simulink model "robot_leg_opt"  (R2015b)
settings: Solver=ode23t  StartTime=0.0  StopTime=2  MaxStep=0.05  RelTol=1e-3
values from neighbouring files (symbols this model uses):
  B0 = q(3)    [costFunc.m]    (also in leg_mechanical_params.m = 3266.28463902)
  DamperStrokeMax = 0.1    [leg_mechanical_params.m]
  dthetaHd = 0    [leg_mechanical_params.m]
  dthetaKd = 0    [leg_mechanical_params.m]
  Hd_knee = 5*0    (= 0)    [leg_mechanical_params.m]
  Hp_knee = 50*0    (= 0)    [leg_mechanical_params.m]
  k_gx = (2*(m_F+m_S+m_T)+m_HAT)*g/0.1    (= 7848)    [leg_mechanical_params.m]
  k_gy = (2*(m_F+m_S+m_T)+m_HAT)*g/0.01    (= 78480)    [leg_mechanical_params.m]
  kap0 = 0    [leg_mechanical_params.m]
  Kd_knee = q(2)    [costFunc.m]    (also in leg_mechanical_params.m = 7.0905816766)
  Kp_knee = q(1)    [costFunc.m]    (also in leg_mechanical_params.m = 4034.50740334)
  LBtnShin = 0    [leg_mechanical_params.m]
  LMidShin = 0    [leg_mechanical_params.m]
  lspring0 = 0.5582    [leg_mechanical_params.m]
  mu_slide = 0.8    [leg_mechanical_params.m]
  mu_stick = 0.9    [leg_mechanical_params.m]
  thetaHd = thetaH0    (= 0.785398163397)    [leg_mechanical_params.m]
  thetaKd = thetaK0    (= -1.0471975512)    [leg_mechanical_params.m]
  v_gx_max = 0.03    [leg_mechanical_params.m]
  v_gy_max = 0.03    [leg_mechanical_params.m]
  vLimit = 0.01    [leg_mechanical_params.m]
  Y0 = 3    [initLegModel.m]
undefined symbols (not defined in the file or in its folder): sgn, t_friction, X, Y, Z
libraries: sm_lib x123, nesl_utility x25, fl_lib x10, simulink x8, simulink_extras x2, dspswit3 x1, HILeg_Lib x1, sm_double_wishbone_suspension_lib x1
(part 1 of 4)
settings Model: Creator=rshum  LastModifiedBy=rshum
settings DataIOCC: SaveFormat=Array
settings DebuggingCC: SolverPrmCheckMsg=warning
settings HardwareCC: ProdBitPerPointer=32  ProdLargestAtomicFloat=None  ProdIntDivRoundTo=Undefined  ProdEndianess=Unspecified  ProdWordSize=32  ProdHWDeviceType=32-bit Generic
settings GRTTargetCC: GeneratePreprocessorConditionals=Disable all
settings ConfigComp: CovModelRefEnable=Off  CovSFcnEnable=off

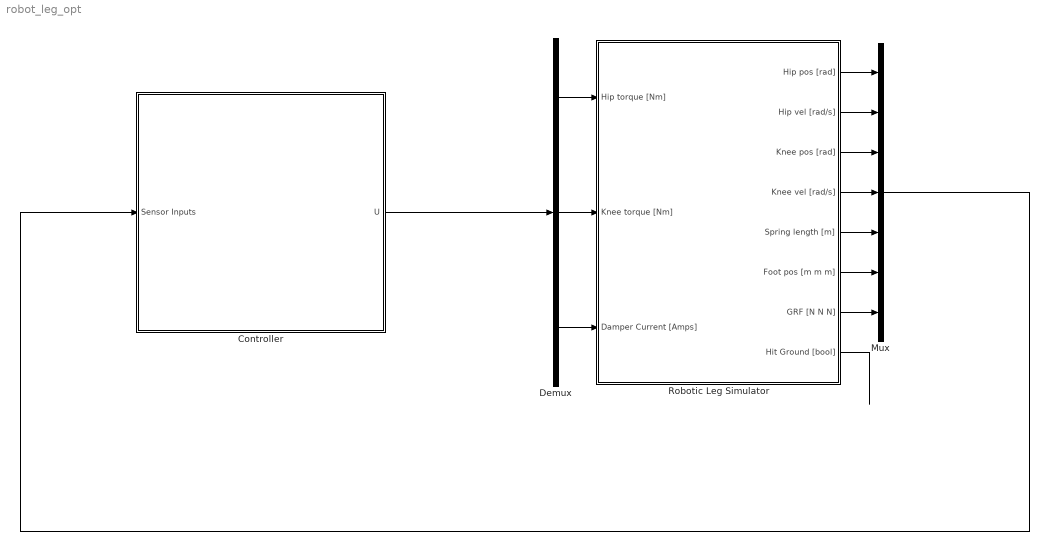
== system robot_leg_opt ==
  Controller : Subsystem
  Demux : Demux  Outputs=3
  Mux : Mux  Inputs=7
  Robotic Leg Simulator : Subsystem
  wires:
  Robotic Leg Simulator/5(Spring length [m]) -> Mux/5
  Demux/3 -> Robotic Leg Simulator/3(Damper Current [Amps])
  Robotic Leg Simulator/1(Hip pos [rad]) -> Mux/1
  Robotic Leg Simulator/2(Hip vel [rad/s]) -> Mux/2
  Robotic Leg Simulator/3(Knee pos [rad]) -> Mux/3
  Robotic Leg Simulator/4(Knee vel [rad/s]) -> Mux/4
  Mux/1 -> Controller/1(Sensor Inputs)
  Demux/1 -> Robotic Leg Simulator/1(Hip torque [Nm])
  Demux/2 -> Robotic Leg Simulator/2(Knee torque [Nm])
  Controller/1(U) -> Demux/1
  Robotic Leg Simulator/6(Foot pos [m m m]) -> Mux/6
  Robotic Leg Simulator/7(GRF [N N N]) -> Mux/7
  Robotic Leg Simulator/8(Hit Ground [bool]) -> ?

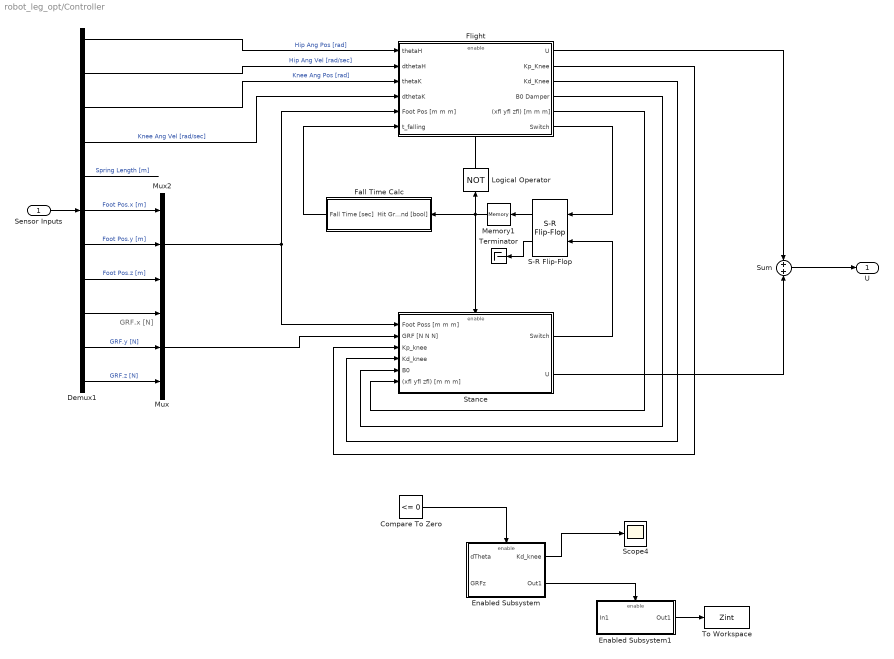
== system robot_leg_opt/Controller ==
  note: GRF.x
      | [N]
  Sensor Inputs : Inport
  Compare To Zero : simulink/Logic and Bit Operations/Compare To Zero  relop=<=  OutDataTypeStr=boolean
  Demux1 : Demux  Outputs=11
  Enabled Subsystem : Subsystem  TreatAsAtomicUnit=on
  Enabled Subsystem1 : Subsystem  TreatAsAtomicUnit=on
  Fall Time Calc : Subsystem
  Flight : Subsystem  TreatAsAtomicUnit=on
  Logical Operator : Logic  Operator=NOT  AllPortsSameDT=off  OutDataTypeStr=boolean
  Memory1 : Memory  X0=1
  Mux : Mux  Inputs=3
  Mux2 : Mux  Inputs=3
  S-R Flip-Flop : simulink_extras/Flip Flops/S-R Flip-Flop  initial_condition=1
  Scope4 : Scope
  Stance : Subsystem  TreatAsAtomicUnit=on
  Sum : Sum
  Terminator : Terminator
  To Workspace : ToWorkspace  VariableName=Zint  SampleTime=-1
      settings: MaxDataPoints=1
  U : Outport
  wires:
  Sensor Inputs/1 -> Demux1/1
  Compare To Zero/1 -> Enabled Subsystem/Enable
  Enabled Subsystem/1(Kd_knee) -> Scope4/1
  Mux/1 -> Stance/2(GRF [N N N])
  Demux1/11 -> Mux/3  "GRF.z [N]"
  Demux1/10 -> Mux/2  "GRF.y [N]"
  Demux1/9 -> Mux/1
  Enabled Subsystem/2(Out1) -> Enabled Subsystem1/Enable
  Enabled Subsystem1/1(Out1) -> To Workspace/1
  Flight/6(Switch) -> S-R Flip-Flop/1
  S-R Flip-Flop/1 -> Memory1/1
  Memory1/1 -> Stance/Enable, Fall Time Calc/1(Hit Ground [bool]), Logical Operator/1
  Stance/1(Switch) -> S-R Flip-Flop/2
  S-R Flip-Flop/2 -> Terminator/1
  Logical Operator/1 -> Flight/Enable
  Mux2/1 -> Flight/5(Foot Pos [m m m]), Stance/1(Foot Poss [m m m])
  Demux1/2 -> Flight/2(dthetaH)  "Hip Ang Vel [rad/sec]"
  Demux1/1 -> Flight/1(thetaH)  "Hip Ang Pos [rad]"
  Demux1/8 -> Mux2/3  "Foot Pos.z [m]"
  Demux1/7 -> Mux2/2  "Foot Pos.y [m]"
  Demux1/6 -> Mux2/1  "Foot Pos.x [m]"
  Demux1/5 -> ?  "Spring Length [m]"
  Demux1/4 -> Flight/4(dthetaK)  "Knee Ang Vel [rad/sec]"
  Demux1/3 -> Flight/3(thetaK)  "Knee Ang Pos [rad]"
  Fall Time Calc/1(Fall Time [sec]) -> Flight/6(t_falling)
  Flight/5((xfl yfl zfl) [m m m]) -> Stance/6((xfl yfl zfl) [m m m])
  Flight/4(B0 Damper) -> Stance/5(B0)
  Flight/3(Kd_Knee) -> Stance/4(Kd_knee)
  Flight/2(Kp_Knee) -> Stance/3(Kp_knee)
  Sum/1 -> U/1
  Flight/1(U) -> Sum/1
  Stance/2(U) -> Sum/2

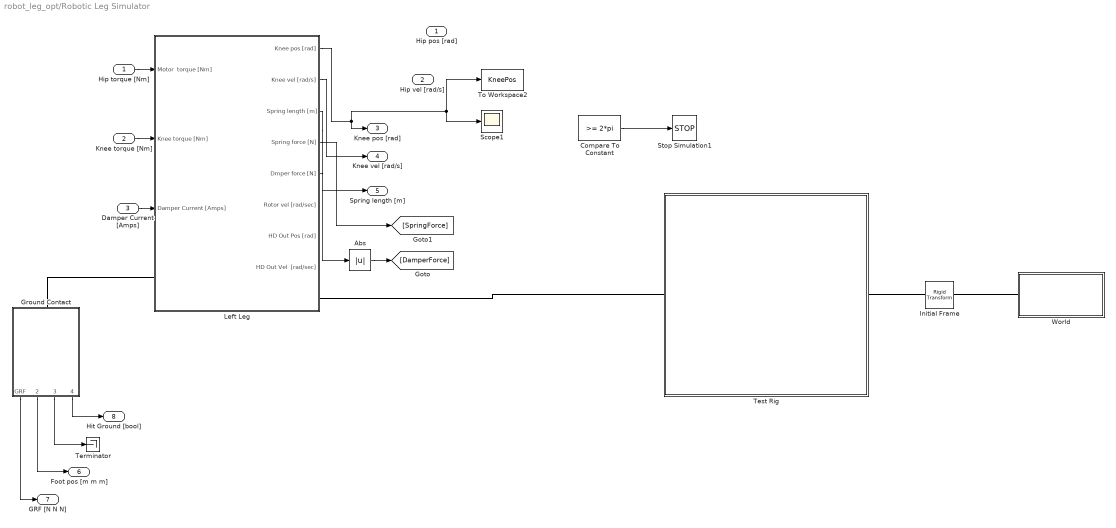
== system robot_leg_opt/Robotic Leg Simulator ==
  Hip torque [Nm] : Inport
  Knee torque [Nm] : Inport  Port=2
  Damper Current [Amps] : Inport  Port=3
  Abs : Abs
  Compare To Constant : simulink/Logic and Bit Operations/Compare To Constant  relop=>=  const=2*pi  OutDataTypeStr=boolean
  Ground Contact : Subsystem  AncestorBlock=HILeg_Lib/Ground Contact  SystemSampleTime=t_friction
  Initial Frame : sm_lib/Frames and Transforms/Rigid Transform  TranslationMethod=Cartesian  TranslationLengthUnit=m  TranslationStandardAxis=+Z  TranslationStandardOffset=0  TranslationCartesianOffset=[0 0 0]  TranslationROffset=0  TranslationROffsetUnits=m  TranslationZOffset=0  TranslationZOffsetUnits=m  TranslationThetaOffset=0  TranslationThetaOffsetUnits=deg  RotationMethod=None  RotationAngleUnits=deg  RotationStandardAxis=+Z  RotationAngle=0  RotationArbitraryAxis=[0 0 1]  FollAlignAxisA=+Z  BaseAlignAxisA=+Y  FollAlignAxisB=+X  BaseAlignAxisB=+X  RotationSequenceAxes=FollowerAxes  RotationSequence=XYX  RotationSequenceAngles=[0 0 0]  RotationSequenceAnglesUnits=deg  RotationMatrix=[1 0 0; 0 1 0; 0 0 1]  BlockFunction=simmechanics.library.frames_transforms.rigid_transform
  Left Leg : Subsystem
  Scope1 : Scope
  Stop Simulation1 : Stop
  Terminator : Terminator
  Test Rig : Subsystem
      mask Display:
      | image(imread('Images/test_rig.JPG'))
      | port_label('rconn',1,'fixture')
      | port_label('lconn',1,'ground')
  To Workspace2 : ToWorkspace  VariableName=KneePos  SampleTime=-1
  World : Subsystem
  Hip pos [rad] : Outport
  Hip vel [rad/s] : Outport  Port=2
  Knee pos [rad] : Outport  Port=3
  Knee vel [rad/s] : Outport  Port=4
  Spring length [m] : Outport  Port=5
  Foot pos [m m m] : Outport  Port=6
  GRF [N N N] : Outport  Port=7
  Hit Ground [bool] : Outport  Port=8
  wires:
  Knee torque [Nm]/1 -> Left Leg/2(Knee torque [Nm])
  Left Leg/1(Knee pos [rad]) -> To Workspace2/1, Scope1/1, Knee pos [rad]/1
  Damper Current [Amps]/1 -> Left Leg/3(Damper Current [Amps])
  ? -> Hip vel [rad/s]/1
  Left Leg/3(Spring length [m]) -> Spring length [m]/1
  Hip torque [Nm]/1 -> Left Leg/1(Motor  torque [Nm])
  Left Leg/5(Dmper force [N]) -> Abs/1
  Left Leg/2(Knee vel [rad/s]) -> Knee vel [rad/s]/1
  Compare To Constant/1 -> Stop Simulation1/1
  Ground Contact/2(POS [m,m,m]) -> Foot pos [m m m]/1
  ? -> Hip pos [rad]/1
  Ground Contact/1(GRF) -> GRF [N N N]/1
  Ground Contact/4(Hit Ground [bool]) -> Hit Ground [bool]/1
  Ground Contact/3(Vel [m,m,m]) -> Terminator/1
  Abs/1 -> [DamperForce]
  Left Leg/4(Spring force [N]) -> [SpringForce]
  connections:
  Initial Frame/LConn1 -- World/LConn1
  Test Rig/LConn1 -- Initial Frame/RConn1
  Ground Contact/LConn1 -- Left Leg/LConn1
  Test Rig/RConn1 -- Left Leg/RConn1

== system robot_leg_opt/Controller/Enabled Subsystem ==
  dTheta : Inport
  GRFz : Inport  Port=2
  Enable : EnablePort
  Constant : Constant
  Gain : Gain  Gain=-1/100
  Sum : Sum  Inputs=|++
  Kd_knee : Outport  OutputWhenDisabled=reset  InitialOutput=0
  Out1 : Outport  Port=2  InitialOutput=0
  wires:
  dTheta/1 -> Sum/1
  Sum/1 -> Gain/1
  GRFz/1 -> Sum/2
  Gain/1 -> Kd_knee/1
  Constant/1 -> Out1/1

== system robot_leg_opt/Controller/Enabled Subsystem1 ==
  In1 : Inport
  Enable : EnablePort
  Abs : Abs
  Integrator : Integrator
  Out1 : Outport
  wires:
  In1/1 -> Abs/1
  Integrator/1 -> Out1/1
  Abs/1 -> Integrator/1

== system robot_leg_opt/Controller/Fall Time Calc ==
  Hit Ground [bool] : Inport
  Constant1 : Constant
  Fall time : Scope
  Integrator : Integrator  ExternalReset=either
  Fall Time [sec] : Outport
  wires:
  Constant1/1 -> Integrator/1
  Integrator/1 -> Fall Time [sec]/1, Fall time/1
  Hit Ground [bool]/1 -> Integrator/2

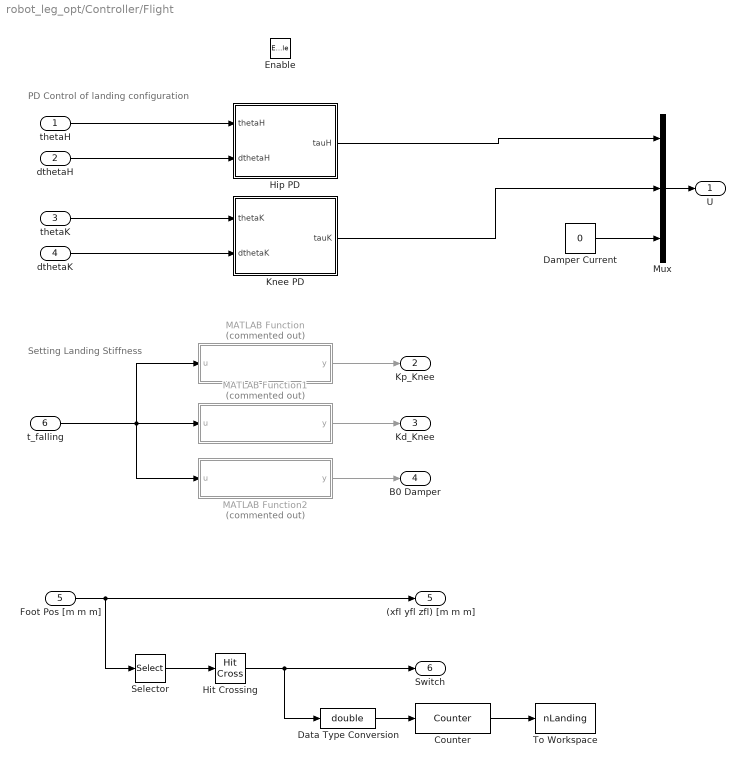
== system robot_leg_opt/Controller/Flight ==
  note: PD Control of landing configuration
  note: Setting Landing Stiffness
  thetaH : Inport
  dthetaH : Inport  Port=2
  thetaK : Inport  Port=3
  dthetaK : Inport  Port=4
  Foot Pos [m m m] : Inport  Port=5
  t_falling : Inport  Port=6
  Enable : EnablePort
  Counter : dspswit3/Counter  Direction=Up  CountEvent=Rising edge  CounterSize=User defined  MaxCount=1e99  InitialCount=0  Output=Count  HitValue=32  ResetInput=off  SamplesPerFrame=1  Ts=1  CntDtype=double  HitDtype=Logical
  Damper Current : Constant  Value=0
  Data Type Conversion : DataTypeConversion  OutDataTypeStr=double
  Hip PD : Subsystem
  Hit Crossing : HitCross  HitCrossingDirection=falling
  Knee PD : Subsystem
  MATLAB Function : MATLAB Function  Commented=on  TreatAsAtomicUnit=on
  MATLAB Function1 : MATLAB Function  Commented=on  TreatAsAtomicUnit=on
  MATLAB Function2 : MATLAB Function  Commented=on  TreatAsAtomicUnit=on
  Mux : Mux  Inputs=3
  Selector : Selector  InputPortWidth=3  IndexOptions=Index vector (dialog)  Indices=[3]  OutputSizes=1
  To Workspace : ToWorkspace  VariableName=nLanding  SampleTime=-1
      settings: MaxDataPoints=1
  U : Outport  OutputWhenDisabled=reset  InitialOutput=[0 0 0]
  Kp_Knee : Outport  Port=2
  Kd_Knee : Outport  Port=3
  B0 Damper : Outport  Port=4
  (xfl yfl zfl) [m m m] : Outport  Port=5
  Switch : Outport  Port=6
  wires:
  MATLAB Function/1(y) -> Kp_Knee/1
  MATLAB Function1/1(y) -> Kd_Knee/1
  MATLAB Function2/1(y) -> B0 Damper/1
  t_falling/1 -> MATLAB Function2/1(u), MATLAB Function/1(u), MATLAB Function1/1(u)
  Hit Crossing/1 -> Data Type Conversion/1, Switch/1
  Data Type Conversion/1 -> Counter/1
  Counter/1 -> To Workspace/1
  Foot Pos [m m m]/1 -> Selector/1, (xfl yfl zfl) [m m m]/1
  Selector/1 -> Hit Crossing/1
  Mux/1 -> U/1
  Hip PD/1(tauH) -> Mux/1
  Knee PD/1(tauK) -> Mux/2
  Damper Current/1 -> Mux/3
  thetaK/1 -> Knee PD/1(thetaK)
  dthetaK/1 -> Knee PD/2(dthetaK)
  thetaH/1 -> Hip PD/1(thetaH)
  dthetaH/1 -> Hip PD/2(dthetaH)

== system robot_leg_opt/Controller/Stance ==
  Foot Poss [m m m] : Inport
  GRF [N N N] : Inport  Port=2
  Kp_knee : Inport  Port=3
  Kd_knee : Inport  Port=4
  B0 : Inport  Port=5
  (xfl yfl zfl) [m m m] : Inport  Port=6
  Enable : EnablePort
  Hit Crossing : HitCross  HitCrossingDirection=falling
  Selector : Selector  InputPortWidth=3  IndexOptions=Index vector (dialog)  Indices=[3]  OutputSizes=1
  Switch : Outport
  U : Outport  Port=2  OutputWhenDisabled=reset  InitialOutput=[0 0 0]
  wires:
  Kp_knee/1 -> U/1
  Selector/1 -> Hit Crossing/1
  Hit Crossing/1 -> Switch/1
  GRF [N N N]/1 -> Selector/1

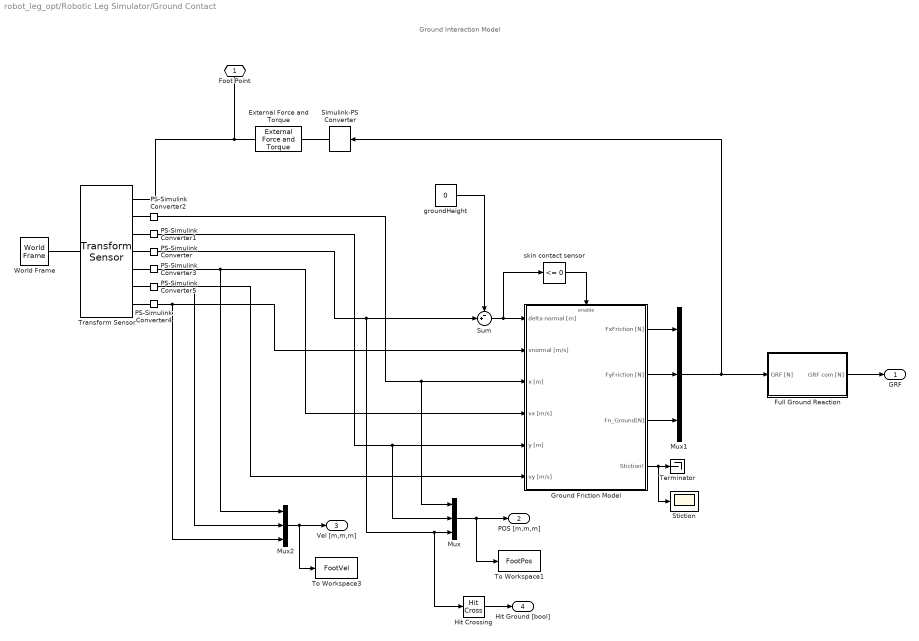
== system robot_leg_opt/Robotic Leg Simulator/Ground Contact ==
  note: Ground Interaction Model
  External Force and Torque : sm_lib/Forces and Torques/External Force and Torque  ForceResolutionFrame=World  EnableForceX=off  EnableForceY=off  EnableForceZ=off  EnableForce=on  TorqueResolutionFrame=AttachedFrame  EnableTorqueX=off  EnableTorqueY=off  EnableTorqueZ=off  EnableTorque=off  BlockFunction=simmechanics.library.forces_torques.external_force_torque
  Full Ground Reaction : Subsystem
  Ground Friction Model : Subsystem
  Hit Crossing : HitCross  HitCrossingDirection=falling
  Mux : Mux  Inputs=3
  Mux1 : Mux  Inputs=3
  Mux2 : Mux  Inputs=3
  PS-Simulink Converter{,1..5} (6 alike) : nesl_utility/PS-Simulink Converter  PhysicalDomain=network_engine_domain  SubClassName=ps_output  LeftPortType=input  RightPortType=output  PseudoPeriodic=off  Frequencies=[]  Unit=1  AffineConversion=off
  Simulink-PS Converter : nesl_utility/Simulink-PS Converter  PhysicalDomain=network_engine_domain  SubClassName=ps_input  LeftPortType=input  RightPortType=output  PseudoPeriodic=off  Frequencies=[]  NoiseDistribution=none  NoiseParameters=[]  Unit=1  AffineConversion=off  InputFiltering=off  SimscapeFilterOrder=1  InputFilterTimeConstant=0.001  UdotUserProvided=1
  Stiction : Scope
  Sum : Sum  Inputs=-+|
  Terminator : Terminator
  To Workspace1 : ToWorkspace  VariableName=FootPos  SampleTime=-1
  To Workspace3 : ToWorkspace  VariableName=FootVel  SampleTime=-1
  Transform Sensor : sm_lib/Frames and Transforms/Transform Sensor  MeasurementFrame=World  SenseAngle=off  SenseAxis=off  SenseAngle1=off  SenseAngle2=off  SenseAngle3=off  SenseQ=off  SenseR=off  SenseOmegaX=off  SenseOmegaY=off  SenseOmegaZ=off  SenseOmega1=off  SenseOmega2=off  SenseOmega3=off  SenseQDot=off  SenseRDot=off  SenseAlphaX=off  SenseAlphaY=off  SenseAlphaZ=off  SenseAlpha1=off  SenseAlpha2=off  SenseAlpha3=off  SenseQDDot=off  SenseRDDot=off  SenseX=on  SenseY=on  SenseZ=on  SenseRad=off  SenseAzim=off  SenseDist=off  SenseInc=off  SenseXDot=on  SenseYDot=on  SenseZDot=on  SenseRadDot=off  SenseAzimDot=off  SenseDistDot=off  SenseIncDot=off  SenseXDDot=off  SenseYDDot=off  SenseZDDot=off  SenseRadDDot=off  SenseAzimDDot=off  SenseDistDDot=off  SenseIncDDot=off  BlockFunction=simmechanics.library.frames_transforms.transform_sensor
  World Frame : sm_lib/Frames and Transforms/World Frame  BlockFunction=simmechanics.library.frames_transforms.world_frame
  groundHeight : Constant  Value=0
  skin contact sensor : simulink/Logic and Bit Operations/Compare To Zero  relop=<=  OutDataTypeStr=boolean
  Foot Point : PMIOPort  Port=1  Side=Left
  GRF : Outport
  POS [m,m,m] : Outport  Port=2
  Vel [m,m,m] : Outport  Port=3
  Hit Ground [bool] : Outport  Port=4
  wires:
  Ground Friction Model/3(Fn_Ground[N]) -> Mux1/3
  Ground Friction Model/2(FyFriction [N]) -> Mux1/2
  PS-Simulink Converter5/1 -> Mux2/2, Ground Friction Model/6(vy [m/s])
  skin contact sensor/1 -> Ground Friction Model/Enable
  groundHeight/1 -> Sum/1
  PS-Simulink Converter4/1 -> Mux2/3, Ground Friction Model/2(vnormal [m/s])
  PS-Simulink Converter3/1 -> Mux2/1, Ground Friction Model/4(vx [m/s])
  PS-Simulink Converter2/1 -> Mux/1, Ground Friction Model/3(x [m])
  PS-Simulink Converter1/1 -> Mux/2, Ground Friction Model/5(y [m])
  Ground Friction Model/4(Stiction!) -> Terminator/1, Stiction/1
  Ground Friction Model/1(FxFriction [N]) -> Mux1/1
  Sum/1 -> Ground Friction Model/1(delta normal [m]), skin contact sensor/1
  Mux/1 -> To Workspace1/1, POS [m,m,m]/1
  Mux2/1 -> To Workspace3/1, Vel [m,m,m]/1
  Mux1/1 -> Simulink-PS Converter/1, Full Ground Reaction/1(GRF [N])
  Full Ground Reaction/1(GRF com [N]) -> GRF/1
  PS-Simulink Converter/1 -> Hit Crossing/1, Mux/3, Sum/2
  Hit Crossing/1 -> Hit Ground [bool]/1
  connections:
  World Frame/RConn1 -- Transform Sensor/LConn1
  Transform Sensor/RConn7 -- PS-Simulink Converter4/LConn1
  Transform Sensor/RConn6 -- PS-Simulink Converter5/LConn1
  PS-Simulink Converter3/LConn1 -- Transform Sensor/RConn5
  PS-Simulink Converter2/LConn1 -- Transform Sensor/RConn2
  Transform Sensor/RConn4 -- PS-Simulink Converter/LConn1
  Transform Sensor/RConn3 -- PS-Simulink Converter1/LConn1
  External Force and Torque/LConn1 -- Simulink-PS Converter/RConn1
  Foot Point/RConn1 -- Transform Sensor/RConn1 -- External Force and Torque/RConn1

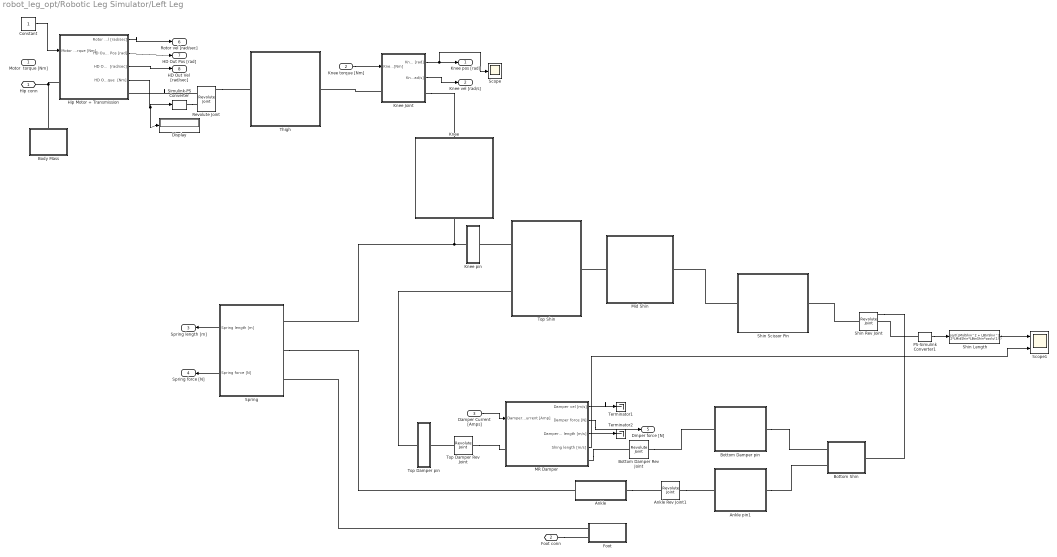
== system robot_leg_opt/Robotic Leg Simulator/Left Leg ==
  Motor  torque [Nm] : Inport
  Knee torque [Nm] : Inport  Port=2
  Damper Current [Amps] : Inport  Port=3
  Ankle : Subsystem
  Ankle Rev Joint1 : sm_lib/Joints/Revolute Joint  SenseConstraintForce=off  SenseConstraintForceX=off  SenseConstraintForceY=off  SenseConstraintForceZ=off  SenseConstraintTorque=off  SenseConstraintTorqueX=off  SenseConstraintTorqueY=off  SenseConstraintTorqueZ=off  SenseTotalForce=off  SenseTotalForceX=off  SenseTotalForceY=off  SenseTotalForceZ=off  SenseTotalTorque=off  SenseTotalTorqueX=off  SenseTotalTorqueY=off  SenseTotalTorqueZ=off  CompositeWrenchDir=FollowerOnBase  CompositeWrenchFrame=BaseFrame  EquilibriumPosition=0  EquilibriumPositionUnits=rad  SpringStiffness=0  SpringStiffnessUnits=m*N/rad  DampingCoefficient=0  DampingCoefficientUnits=m*s*N/rad  TorqueActuationMode=NoTorque  MotionActuationMode=ComputedMotion  SensePosition=off  SenseVelocity=off  SenseAcceleration=off  SenseTorqueForce=off  PositionTargetSpecify=off  PositionTargetPriority=Low  PositionTargetValue=-30  PositionTargetValueUnits=deg  VelocityTargetSpecify=off  VelocityTargetPriority=High  VelocityTargetValue=0  VelocityTargetValueUnits=deg/s  BlockFunction=simmechanics.library.joints.revolute_joint
  Ankle pin1 : Subsystem
  Body Mass : Subsystem
  Bottom Damper Rev Joint : sm_lib/Joints/Revolute Joint  SenseConstraintForce=off  SenseConstraintForceX=off  SenseConstraintForceY=off  SenseConstraintForceZ=off  SenseConstraintTorque=off  SenseConstraintTorqueX=off  SenseConstraintTorqueY=off  SenseConstraintTorqueZ=off  SenseTotalForce=off  SenseTotalForceX=off  SenseTotalForceY=off  SenseTotalForceZ=off  SenseTotalTorque=off  SenseTotalTorqueX=off  SenseTotalTorqueY=off  SenseTotalTorqueZ=off  CompositeWrenchDir=FollowerOnBase  CompositeWrenchFrame=BaseFrame  EquilibriumPosition=0  EquilibriumPositionUnits=rad  SpringStiffness=0  SpringStiffnessUnits=m*N/rad  DampingCoefficient=0  DampingCoefficientUnits=m*s*N/rad  TorqueActuationMode=NoTorque  MotionActuationMode=ComputedMotion  SensePosition=off  SenseVelocity=off  SenseAcceleration=off  SenseTorqueForce=off  PositionTargetSpecify=off  PositionTargetPriority=Low  PositionTargetValue=-30  PositionTargetValueUnits=deg  VelocityTargetSpecify=off  VelocityTargetPriority=High  VelocityTargetValue=0  VelocityTargetValueUnits=deg/s  BlockFunction=simmechanics.library.joints.revolute_joint
  Bottom Damper pin : Subsystem
  Bottom Shin : Subsystem
  Constant : Constant
  Display : Display
  "Foot " : Subsystem
  Hip Motor + Transmission : Subsystem
  Knee : Subsystem
      mask Display:
      | image(imread('Images/knee.JPG'))
      | port_label('lconn',1,'Knee-Thigh conn')
      | port_label('rconn',1,'pin')
  Knee Joint : Subsystem
  Knee pin : Subsystem
      mask Display: image(imread('knee_closure_pin.JPG'))
  MR Damper : Subsystem
  "Mid Shin " : Subsystem
  PS-Simulink Converter1 : nesl_utility/PS-Simulink Converter  PhysicalDomain=network_engine_domain  SubClassName=ps_output  LeftPortType=input  RightPortType=output  PseudoPeriodic=off  Frequencies=[]  Unit=1  AffineConversion=off
  Revolute Joint : sm_lib/Joints/Revolute Joint  SenseConstraintForce=off  SenseConstraintForceX=off  SenseConstraintForceY=off  SenseConstraintForceZ=off  SenseConstraintTorque=off  SenseConstraintTorqueX=off  SenseConstraintTorqueY=off  SenseConstraintTorqueZ=off  SenseTotalForce=off  SenseTotalForceX=off  SenseTotalForceY=off  SenseTotalForceZ=off  SenseTotalTorque=off  SenseTotalTorqueX=off  SenseTotalTorqueY=off  SenseTotalTorqueZ=off  CompositeWrenchDir=FollowerOnBase  CompositeWrenchFrame=BaseFrame  EquilibriumPosition=0  EquilibriumPositionUnits=deg  SpringStiffness=0  SpringStiffnessUnits=N*m/deg  DampingCoefficient=0  DampingCoefficientUnits=N*m/(deg/s)  TorqueActuationMode=InputTorque  MotionActuationMode=ComputedMotion  SensePosition=on  SenseVelocity=on  SenseAcceleration=on  SenseTorqueForce=off  PositionTargetSpecify=on  PositionTargetPriority=High  PositionTargetValue=thetaH0  PositionTargetValueUnits=rad  VelocityTargetSpecify=off  VelocityTargetPriority=High  VelocityTargetValue=0  VelocityTargetValueUnits=deg/s  BlockFunction=simmechanics.library.joints.revolute_joint
  Scope : Scope
  Scope1 : Scope  NumInputPorts=2
  Shin Length : Fcn  Expr=sqrt(LMidShin^2 + LBtnShin^2 - 2*LMidShin*LBtnShin*cos(u(1)))
  Shin Rev Joint : sm_lib/Joints/Revolute Joint  SenseConstraintForce=off  SenseConstraintForceX=off  SenseConstraintForceY=off  SenseConstraintForceZ=off  SenseConstraintTorque=off  SenseConstraintTorqueX=off  SenseConstraintTorqueY=off  SenseConstraintTorqueZ=off  SenseTotalForce=off  SenseTotalForceX=off  SenseTotalForceY=off  SenseTotalForceZ=off  SenseTotalTorque=off  SenseTotalTorqueX=off  SenseTotalTorqueY=off  SenseTotalTorqueZ=off  CompositeWrenchDir=FollowerOnBase  CompositeWrenchFrame=BaseFrame  EquilibriumPosition=0  EquilibriumPositionUnits=rad  SpringStiffness=0  SpringStiffnessUnits=m*N/rad  DampingCoefficient=0  DampingCoefficientUnits=m*s*N/rad  TorqueActuationMode=NoTorque  MotionActuationMode=ComputedMotion  SensePosition=on  SenseVelocity=on  SenseAcceleration=off  SenseTorqueForce=off  PositionTargetSpecify=on  PositionTargetPriority=Low  PositionTargetValue=-35  PositionTargetValueUnits=deg  VelocityTargetSpecify=off  VelocityTargetPriority=High  VelocityTargetValue=0  VelocityTargetValueUnits=deg/s  BlockFunction=simmechanics.library.joints.revolute_joint
  Shin Scissor Pin : Subsystem
  Simulink-PS Converter : nesl_utility/Simulink-PS Converter  PhysicalDomain=network_engine_domain  SubClassName=ps_input  LeftPortType=input  RightPortType=output  PseudoPeriodic=off  Frequencies=[]  NoiseDistribution=none  NoiseParameters=[]  Unit=1  AffineConversion=off  InputFiltering=off  SimscapeFilterOrder=1  InputFilterTimeConstant=0.001  UdotUserProvided=1
  Spring : Subsystem
  Terminator1 : Terminator
  Terminator2 : Terminator
  Thigh : Subsystem
  Top Damper Rev Joint : sm_lib/Joints/Revolute Joint  SenseConstraintForce=off  SenseConstraintForceX=off  SenseConstraintForceY=off  SenseConstraintForceZ=off  SenseConstraintTorque=off  SenseConstraintTorqueX=off  SenseConstraintTorqueY=off  SenseConstraintTorqueZ=off  SenseTotalForce=off  SenseTotalForceX=off  SenseTotalForceY=off  SenseTotalForceZ=off  SenseTotalTorque=off  SenseTotalTorqueX=off  SenseTotalTorqueY=off  SenseTotalTorqueZ=off  CompositeWrenchDir=FollowerOnBase  CompositeWrenchFrame=BaseFrame  EquilibriumPosition=0  EquilibriumPositionUnits=rad  SpringStiffness=0  SpringStiffnessUnits=m*N/rad  DampingCoefficient=0  DampingCoefficientUnits=m*s*N/rad  TorqueActuationMode=NoTorque  MotionActuationMode=ComputedMotion  SensePosition=off  SenseVelocity=off  SenseAcceleration=off  SenseTorqueForce=off  PositionTargetSpecify=off  PositionTargetPriority=Low  PositionTargetValue=-30  PositionTargetValueUnits=deg  VelocityTargetSpecify=off  VelocityTargetPriority=High  VelocityTargetValue=0  VelocityTargetValueUnits=deg/s  BlockFunction=simmechanics.library.joints.revolute_joint
  Top Damper pin : Subsystem
      mask Display: image(imread('knee_closure_pin.JPG'))
  Top Shin : Subsystem
  Hip conn : PMIOPort  Port=1  Side=Right
  Foot conn : PMIOPort  Port=2  Side=Left
  Knee pos [rad] : Outport
  Knee vel [rad/s] : Outport  Port=2
  Spring length [m] : Outport  Port=3
  Spring force [N] : Outport  Port=4
  Dmper force [N] : Outport  Port=5
  Rotor vel [rad/sec] : Outport  Port=6
  HD Out Pos [rad] : Outport  Port=7
  HD Out Vel  [rad/sec] : Outport  Port=8
  wires:
  Knee Joint/1(Knee pos [rad]) -> Scope/1, Knee pos [rad]/1
  Knee Joint/2(Knee vel [rad/s]) -> Knee vel [rad/s]/1
  Damper Current [Amps]/1 -> MR Damper/1(Damper current [Amp])
  Knee torque [Nm]/1 -> Knee Joint/1(Knee Torque [Nm])
  Spring/1(Spring length [m]) -> Spring length [m]/1
  Spring/2(Spring force [N]) -> Spring force [N]/1
  MR Damper/2(Damper force [N]) -> Dmper force [N]/1
  MR Damper/1(Damper vel [m/s]) -> Terminator1/1
  PS-Simulink Converter1/1 -> Shin Length/1
  Shin Length/1 -> Scope1/1
  MR Damper/4(Shing length [m/s]) -> Scope1/2
  MR Damper/3(Damper length [m/s]) -> Terminator2/1
  Hip Motor + Transmission/4(HD Out Torque  [Nm]) -> Display/1, Simulink-PS Converter/1
  Hip Motor + Transmission/2(HD Out Pos [rad]) -> HD Out Pos [rad]/1
  Hip Motor + Transmission/1(Rotor vel [rad/sec]) -> Rotor vel [rad/sec]/1
  Hip Motor + Transmission/3(HD Out Vel  [rad/sec]) -> HD Out Vel  [rad/sec]/1
  Constant/1 -> Hip Motor + Transmission/1(Motor torque [Nm])
  connections:
  Knee pin/LConn1 -- Spring/LConn1 -- Knee/RConn1
  Top Shin/RConn1 -- Knee pin/RConn1
  Top Damper Rev Joint/LConn1 -- Top Damper pin/RConn1
  Top Damper Rev Joint/RConn1 -- MR Damper/LConn1
  Foot conn/RConn1 -- "Foot "/RConn2
  "Mid Shin "/RConn1 -- Top Shin/LConn1
  Shin Rev Joint/RConn1 -- Bottom Shin/LConn1
  Shin Rev Joint/LConn1 -- Shin Scissor Pin/RConn1
  Shin Scissor Pin/LConn1 -- "Mid Shin "/LConn1
  Ankle Rev Joint1/LConn1 -- Ankle pin1/RConn1
  Bottom Damper pin/LConn1 -- Bottom Shin/RConn1
  Ankle pin1/LConn1 -- Bottom Shin/RConn2
  Ankle/LConn1 -- Ankle Rev Joint1/RConn1
  Bottom Damper Rev Joint/LConn1 -- Bottom Damper pin/RConn1
  Bottom Damper Rev Joint/RConn1 -- MR Damper/RConn1
  Top Shin/RConn2 -- Top Damper pin/LConn1
  Hip Motor + Transmission/LConn1 -- Body Mass/RConn1 -- Hip conn/RConn1
  Spring/LConn2 -- Ankle/RConn1
  "Foot "/RConn1 -- Spring/LConn3
  Knee Joint/RConn1 -- Knee/LConn1
  Knee Joint/LConn1 -- Thigh/LConn1
  PS-Simulink Converter1/LConn1 -- Shin Rev Joint/RConn2
  Revolute Joint/RConn1 -- Thigh/RConn1
  Revolute Joint/LConn1 -- Hip Motor + Transmission/RConn1
  Simulink-PS Converter/RConn1 -- Revolute Joint/LConn2

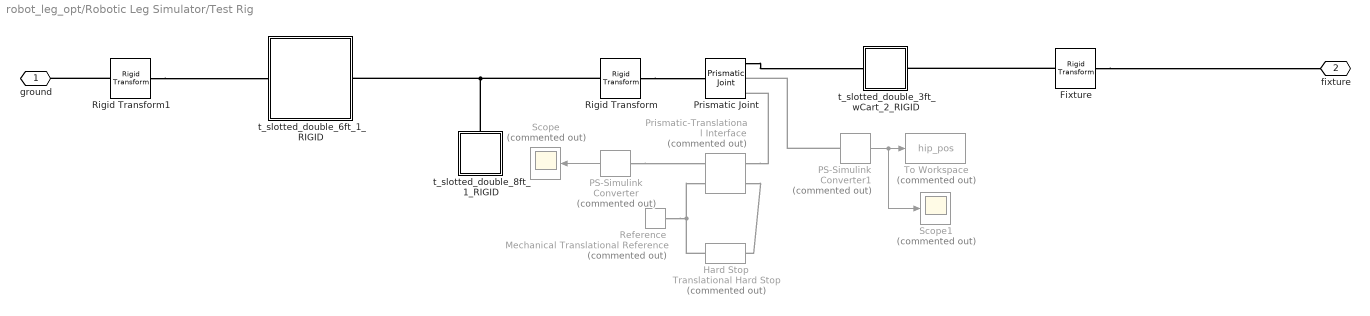
== system robot_leg_opt/Robotic Leg Simulator/Test Rig ==
  Fixture : sm_lib/Frames and Transforms/Rigid Transform  TranslationMethod=None  TranslationLengthUnit=m  TranslationStandardAxis=+Z  TranslationStandardOffset=0  TranslationCartesianOffset=[0 0 0]  TranslationROffset=0  TranslationROffsetUnits=m  TranslationZOffset=0  TranslationZOffsetUnits=m  TranslationThetaOffset=0  TranslationThetaOffsetUnits=deg  RotationMethod=None  RotationAngleUnits=deg  RotationStandardAxis=+X  RotationAngle=-90  RotationArbitraryAxis=[0 0 1]  FollAlignAxisA=+X  BaseAlignAxisA=+Y  FollAlignAxisB=+Y  BaseAlignAxisB=+Z  RotationSequenceAxes=FollowerAxes  RotationSequence=XYX  RotationSequenceAngles=[0 0 0]  RotationSequenceAnglesUnits=deg  RotationMatrix=[1 0 0; 0 1 0; 0 0 1]  BlockFunction=simmechanics.library.frames_transforms.rigid_transform
  Hard Stop : fl_lib/Mechanical/Translational Elements/Translational Hard Stop  Commented=on  upper_bnd=Y0*50 m  lower_bnd=-Y0*50 m  stiff_up=2e6 N/m  stiff_low=2e6 N/m  D_up=150 N/(m/s)  D_low=150 N/(m/s)  v_specify=off  v_priority=High  v=0 m/s  f_specify=off  f_priority=High  f=0 N  x_specify=on  x_priority=High  x=1 cm
  PS-Simulink Converter : nesl_utility/PS-Simulink Converter  Commented=on  PhysicalDomain=network_engine_domain  SubClassName=ps_output  LeftPortType=input  RightPortType=output  PseudoPeriodic=off  Frequencies=[]  Unit=N  AffineConversion=off
  PS-Simulink Converter1 : nesl_utility/PS-Simulink Converter  Commented=on  PhysicalDomain=network_engine_domain  SubClassName=ps_output  LeftPortType=input  RightPortType=output  PseudoPeriodic=off  Frequencies=[]  Unit=1  AffineConversion=off
  Prismatic Joint : sm_lib/Joints/Prismatic Joint  SenseConstraintForce=off  SenseConstraintForceX=off  SenseConstraintForceY=off  SenseConstraintForceZ=off  SenseConstraintTorque=off  SenseConstraintTorqueX=off  SenseConstraintTorqueY=off  SenseConstraintTorqueZ=off  SenseTotalForce=off  SenseTotalForceX=off  SenseTotalForceY=off  SenseTotalForceZ=off  SenseTotalTorque=off  SenseTotalTorqueX=off  SenseTotalTorqueY=off  SenseTotalTorqueZ=off  CompositeWrenchDir=FollowerOnBase  CompositeWrenchFrame=BaseFrame  EquilibriumPosition=0  EquilibriumPositionUnits=m  SpringStiffness=0  SpringStiffnessUnits=N/m  DampingCoefficient=0  DampingCoefficientUnits=N/(m/s)  TorqueActuationMode=NoTorque  MotionActuationMode=ComputedMotion  SensePosition=on  SenseVelocity=on  SenseAcceleration=off  SenseTorqueForce=off  PositionTargetSpecify=on  PositionTargetPriority=High  PositionTargetValue=H0  PositionTargetValueUnits=m  VelocityTargetSpecify=off  VelocityTargetPriority=High  VelocityTargetValue=0  VelocityTargetValueUnits=m/s  BlockFunction=simmechanics.library.joints.prismatic_joint
  Prismatic-Translational Interface : sm_double_wishbone_suspension_lib/Testing Platform/Prismatic-Translational Interface  Commented=on
  Reference : fl_lib/Mechanical/Translational Elements/Mechanical Translational Reference  Commented=on
  Rigid Transform : sm_lib/Frames and Transforms/Rigid Transform  TranslationMethod=None  TranslationLengthUnit=m  TranslationStandardAxis=+Z  TranslationStandardOffset=0  TranslationCartesianOffset=[0 0 0]  TranslationROffset=0  TranslationROffsetUnits=m  TranslationZOffset=0  TranslationZOffsetUnits=m  TranslationThetaOffset=0  TranslationThetaOffsetUnits=deg  RotationMethod=StandardAxis  RotationAngleUnits=deg  RotationStandardAxis=+X  RotationAngle=-90  RotationArbitraryAxis=[0 0 1]  FollAlignAxisA=+X  BaseAlignAxisA=+Y  FollAlignAxisB=+Y  BaseAlignAxisB=+Z  RotationSequenceAxes=FollowerAxes  RotationSequence=XYX  RotationSequenceAngles=[0 0 0]  RotationSequenceAnglesUnits=deg  RotationMatrix=[1 0 0; 0 1 0; 0 0 1]  BlockFunction=simmechanics.library.frames_transforms.rigid_transform
  Rigid Transform1 : sm_lib/Frames and Transforms/Rigid Transform  TranslationMethod=Cartesian  TranslationLengthUnit=m  TranslationStandardAxis=+Z  TranslationStandardOffset=0  TranslationCartesianOffset=[0 0.5 0]  TranslationROffset=0  TranslationROffsetUnits=m  TranslationZOffset=0  TranslationZOffsetUnits=m  TranslationThetaOffset=0  TranslationThetaOffsetUnits=deg  RotationMethod=AlignedAxes  RotationAngleUnits=deg  RotationStandardAxis=+X  RotationAngle=90  RotationArbitraryAxis=[0 0 1]  FollAlignAxisA=+Y  BaseAlignAxisA=+Z  FollAlignAxisB=+X  BaseAlignAxisB=-Y  RotationSequenceAxes=FollowerAxes  RotationSequence=XYX  RotationSequenceAngles=[0 0 0]  RotationSequenceAnglesUnits=deg  RotationMatrix=[1 0 0; 0 1 0; 0 0 1]  BlockFunction=simmechanics.library.frames_transforms.rigid_transform
  Scope : Scope  Commented=on
  Scope1 : Scope  Commented=on
  To Workspace : ToWorkspace  Commented=on  VariableName=hip_pos  SaveFormat=Timeseries  SampleTime=-1
  t_slotted_double_3ft_wCart_2_RIGID : Subsystem
  t_slotted_double_6ft_1_RIGID : Subsystem
  t_slotted_double_8ft_1_RIGID : Subsystem
  ground : PMIOPort  Port=1  Side=Left
  fixture : PMIOPort  Port=2  Side=Right
  wires:
  PS-Simulink Converter/1 -> Scope/1
  PS-Simulink Converter1/1 -> Scope1/1, To Workspace/1
  connections:
  Prismatic-Translational Interface/LConn1 -- Prismatic Joint/RConn3
  t_slotted_double_8ft_1_RIGID/LConn1 -- Rigid Transform/LConn1 -- t_slotted_double_6ft_1_RIGID/RConn1
  Prismatic Joint/RConn1 -- t_slotted_double_3ft_wCart_2_RIGID/LConn1
  Rigid Transform/RConn1 -- Prismatic Joint/LConn1
  Hard Stop/RConn1 -- Prismatic-Translational Interface/RConn2 -- Reference/LConn1
  Prismatic-Translational Interface/LConn2 -- Hard Stop/LConn1
  PS-Simulink Converter/LConn1 -- Prismatic-Translational Interface/RConn1
  PS-Simulink Converter1/LConn1 -- Prismatic Joint/RConn2
  Rigid Transform1/RConn1 -- t_slotted_double_6ft_1_RIGID/LConn1
  Rigid Transform1/LConn1 -- ground/RConn1
  Fixture/LConn1 -- t_slotted_double_3ft_wCart_2_RIGID/RConn1
  Fixture/RConn1 -- fixture/RConn1

== system robot_leg_opt/Robotic Leg Simulator/World ==
  Ground Tile : Subsystem
  MechanismConfiguration : sm_lib/Utilities/Mechanism Configuration  UniformGravity=Constant  GravityVector=[0 0 0*-9.81]  GravityUnits=m/s^2  LinearizationDelta=0.001  BlockFunction=simmechanics.library.utilities.mechanism_configuration
  Solver Configuration : nesl_utility/Solver Configuration  PhysicalDomain=network_engine_domain  SubClassName=solver  LeftPortType=input  RightPortType=generic  Accelerate=off  Tones=[]  Harmonics=[]  SimulateNoise=off  Profile=off  UseLocalSampling=off  EnableSwitchedLinearOptims=on  FrequencyDomain=off  UseCCode=off  RelTol=0.001  AbsTol=1e-06  MinStep=1e-09  ToWorkspace=off  RevertToSquareIcSolve=off  NumHomotopyIterations=100  PhasorMode=off  PhasorModeNumHarmonics=1  DoDC=off  ResidualTolerance=1e-09  UseLocalSolver=off  LocalSolverChoice=NE_BACKWARD_EULER_ADVANCER  LocalSolverSampleTime=0.001  DoFixedCost=off  MaxNonlinIter=3  MaxModeIter=2  LinearAlgebra=Sparse  DelaysMemoryBudget=1024  AutomaticFiltering=on  FilteringTimeConstant=0.001
  World : sm_lib/Frames and Transforms/World Frame  BlockFunction=simmechanics.library.frames_transforms.world_frame
  Ground conn : PMIOPort  Port=1  Side=Left
  connections:
  World/RConn1 -- Ground Tile/LConn1 -- Ground conn/RConn1 -- Solver Configuration/RConn1 -- MechanismConfiguration/RConn1

== system robot_leg_opt/Controller/Flight/Hip PD ==
  thetaH : Inport
  dthetaH : Inport  Port=2
  Constant : Constant  Value=dthetaHd
  Constant1 : Constant  Value=thetaHd
  Gain : Gain  Gain=Hp_knee
  Gain1 : Gain  Gain=Hd_knee
  Scope : Scope  NumInputPorts=2
  Scope1 : Scope  NumInputPorts=2
  Sum : Sum  Inputs=|-+
  Sum1 : Sum  Inputs=+-|
  Sum2 : Sum
  tauH : Outport
  wires:
  dthetaH/1 -> Sum/1
  Sum/1 -> Gain1/1
  Constant/1 -> Sum/2
  thetaH/1 -> Scope1/2, Sum1/2
  Sum1/1 -> Gain/1
  Gain1/1 -> Scope/2, Sum2/2
  Constant1/1 -> Scope1/1, Sum1/1
  Gain/1 -> Scope/1, Sum2/1
  Sum2/1 -> tauH/1

== system robot_leg_opt/Controller/Flight/Knee PD ==
  thetaK : Inport
  dthetaK : Inport  Port=2
  Constant : Constant  Value=dthetaKd
  Constant1 : Constant  Value=thetaKd
  Gain : Gain  Gain=Kp_knee
  Gain1 : Gain  Gain=Kd_knee
  Scope : Scope  NumInputPorts=2
  Scope1 : Scope  NumInputPorts=2
  Sum : Sum  Inputs=|-+
  Sum1 : Sum  Inputs=+-|
  Sum2 : Sum
  tauK : Outport
  wires:
  dthetaK/1 -> Sum/1
  Sum/1 -> Gain1/1
  Constant/1 -> Sum/2
  thetaK/1 -> Scope1/2, Sum1/2
  Sum1/1 -> Gain/1
  Gain1/1 -> Scope/2, Sum2/2
  Constant1/1 -> Scope1/1, Sum1/1
  Gain/1 -> Scope/1, Sum2/1
  Sum2/1 -> tauK/1

== system robot_leg_opt/Robotic Leg Simulator/Ground Contact/Full Ground Reaction ==
  GRF [N] : Inport
  Mux3 : Mux  Inputs=2
  Scope3 : Scope
  Selector : Selector  InputPortWidth=3  IndexOptions=Index vector (dialog)  Indices=[3]  OutputSizes=1
  Selector1 : Selector  InputPortWidth=3  IndexOptions=Index vector (dialog)  Indices=[1 2]  OutputSizes=1
  Sum2 : Sum  Inputs=+++
  To Workspace : ToWorkspace  VariableName=GRF1  SaveFormat=Timeseries  SampleTime=-1
  GRF com [N] : Outport
  wires:
  Selector/1 -> Sum2/1  "Fn_Ground"
  Sum2/1 -> Mux3/2
  [SpringForce] -> Sum2/3
  Selector1/1 -> Mux3/1
  [DamperForce] -> Sum2/2
  Mux3/1 -> GRF com [N]/1, Scope3/1, To Workspace/1
  GRF [N]/1 -> Selector1/1, Selector/1

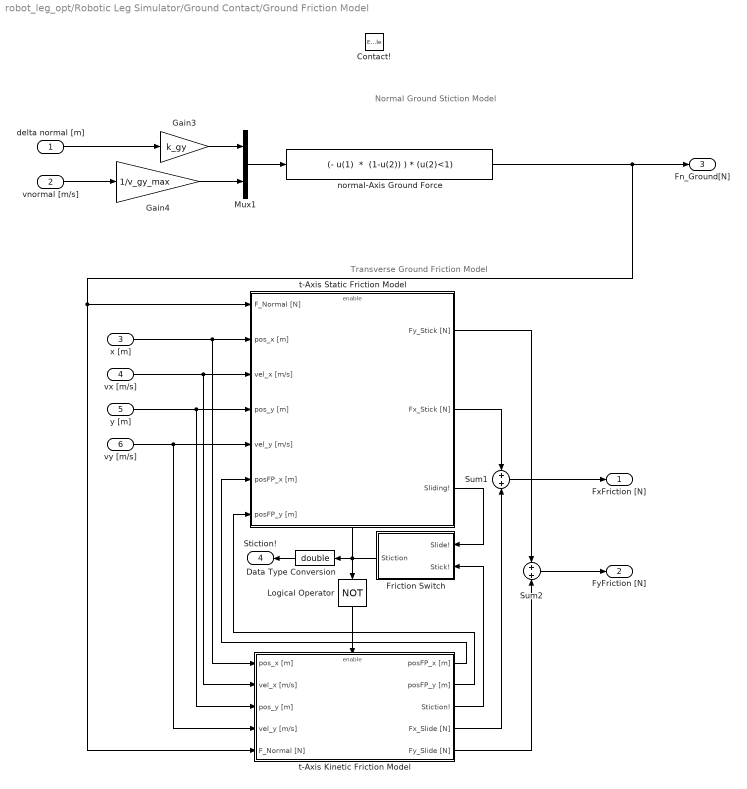
== system robot_leg_opt/Robotic Leg Simulator/Ground Contact/Ground Friction Model ==
  note: Normal Ground Stiction Model
  note: Transverse Ground Friction Model
  delta normal [m] : Inport
  vnormal [m/s] : Inport  Port=2
  x [m] : Inport  Port=3
  vx [m/s] : Inport  Port=4
  y [m] : Inport  Port=5
  vy [m/s] : Inport  Port=6
  Contact! : EnablePort  StatesWhenEnabling=reset
  Data Type Conversion : DataTypeConversion  OutDataTypeStr=double
  Friction Switch : Subsystem
  Gain3 : Gain  Gain=k_gy
  Gain4 : Gain  Gain=1/v_gy_max
  Logical Operator : Logic  Operator=NOT  AllPortsSameDT=off  OutDataTypeStr=boolean
  Mux1 : Mux  Inputs=2
  Sum1 : Sum
  Sum2 : Sum
  normal-Axis Ground Force : Fcn  Expr="(- u(1)  *  (1-u(2)) ) * (u(2)<1)"
  t-Axis Kinetic Friction Model : Subsystem
  t-Axis Static Friction Model : Subsystem
  FxFriction [N] : Outport  OutputWhenDisabled=reset  InitialOutput=0
      settings: AttributesFormatString=initial = '%<InitialOutput>'\nwhen\ndisabled\n'%<OutputWhenDisabled>'
  FyFriction [N] : Outport  Port=2  OutputWhenDisabled=reset  InitialOutput=0
      settings: AttributesFormatString=initial = '%<InitialOutput>'\nwhen\ndisabled\n'%<OutputWhenDisabled>'
  Fn_Ground[N] : Outport  Port=3  OutputWhenDisabled=reset  InitialOutput=0
      settings: AttributesFormatString=initial = '%<InitialOutput>'\nwhen disabled = '%<OutputWhenDisabled>'
  Stiction! : Outport  Port=4  OutputWhenDisabled=reset  InitialOutput=0
      settings: AttributesFormatString=initial = '%<InitialOutput>'\nwhen\ndisabled\n'%<OutputWhenDisabled>'
  wires:
  Data Type Conversion/1 -> Stiction!/1
  vy [m/s]/1 -> t-Axis Static Friction Model/5(vel_y [m/s]), t-Axis Kinetic Friction Model/4(vel_y [m/s])
  y [m]/1 -> t-Axis Kinetic Friction Model/3(pos_y [m]), t-Axis Static Friction Model/4(pos_y [m])
  t-Axis Kinetic Friction Model/2(posFP_y [m]) -> t-Axis Static Friction Model/7(posFP_y [m])
  Sum2/1 -> FyFriction [N]/1
  t-Axis Kinetic Friction Model/5(Fy_Slide [N]) -> Sum2/2
  t-Axis Static Friction Model/1(Fy_Stick [N]) -> Sum2/1
  Gain4/1 -> Mux1/2
  Gain3/1 -> Mux1/1
  Mux1/1 -> normal-Axis Ground Force/1
  Logical Operator/1 -> t-Axis Kinetic Friction Model/Enable
  t-Axis Kinetic Friction Model/3(Stiction!) -> Friction Switch/2(Stick!)
  t-Axis Static Friction Model/3(Sliding!) -> Friction Switch/1(Slide!)
  Friction Switch/1(Stiction) -> t-Axis Static Friction Model/Enable, Logical Operator/1, Data Type Conversion/1
  Sum1/1 -> FxFriction [N]/1
  t-Axis Static Friction Model/2(Fx_Stick [N]) -> Sum1/1
  t-Axis Kinetic Friction Model/4(Fx_Slide [N]) -> Sum1/2
  t-Axis Kinetic Friction Model/1(posFP_x [m]) -> t-Axis Static Friction Model/6(posFP_x [m])
  vx [m/s]/1 -> t-Axis Static Friction Model/3(vel_x [m/s]), t-Axis Kinetic Friction Model/2(vel_x [m/s])
  x [m]/1 -> t-Axis Static Friction Model/2(pos_x [m]), t-Axis Kinetic Friction Model/1(pos_x [m])
  vnormal [m/s]/1 -> Gain4/1
  delta normal [m]/1 -> Gain3/1
  normal-Axis Ground Force/1 -> Fn_Ground[N]/1, t-Axis Kinetic Friction Model/5(F_Normal [N]), t-Axis Static Friction Model/1(F_Normal [N])

== system robot_leg_opt/Robotic Leg Simulator/Left Leg/Ankle ==
  Ref-2-Shin : sm_lib/Frames and Transforms/Rigid Transform  TranslationMethod=Cartesian  TranslationLengthUnit=cm  TranslationStandardAxis=+Z  TranslationStandardOffset=0  TranslationCartesianOffset=[13.96 10.6 -1.1]  TranslationROffset=0  TranslationROffsetUnits=m  TranslationZOffset=0  TranslationZOffsetUnits=m  TranslationThetaOffset=0  TranslationThetaOffsetUnits=deg  RotationMethod=None  RotationAngleUnits=deg  RotationStandardAxis=+Z  RotationAngle=15  RotationArbitraryAxis=[0 0 1]  FollAlignAxisA=+X  BaseAlignAxisA=+Y  FollAlignAxisB=+Y  BaseAlignAxisB=+Z  RotationSequenceAxes=FollowerAxes  RotationSequence=XYX  RotationSequenceAngles=[0 0 0]  RotationSequenceAnglesUnits=deg  RotationMatrix=[1 0 0; 0 1 0; 0 0 1]  BlockFunction=simmechanics.library.frames_transforms.rigid_transform
  Ref-2-Spring : sm_lib/Frames and Transforms/Rigid Transform  TranslationMethod=Cartesian  TranslationLengthUnit=cm  TranslationStandardAxis=+Z  TranslationStandardOffset=0  TranslationCartesianOffset=[-26.7 -18 1.1]  TranslationROffset=0  TranslationROffsetUnits=m  TranslationZOffset=0  TranslationZOffsetUnits=m  TranslationThetaOffset=0  TranslationThetaOffsetUnits=deg  RotationMethod=StandardAxis  RotationAngleUnits=deg  RotationStandardAxis=+Z  RotationAngle=16.9  RotationArbitraryAxis=[0 0 1]  FollAlignAxisA=+X  BaseAlignAxisA=+Y  FollAlignAxisB=+Y  BaseAlignAxisB=+Z  RotationSequenceAxes=FollowerAxes  RotationSequence=XYX  RotationSequenceAngles=[0 0 0]  RotationSequenceAnglesUnits=deg  RotationMatrix=[1 0 0; 0 1 0; 0 0 1]  BlockFunction=simmechanics.library.frames_transforms.rigid_transform
  Ref-2-Spring2 : sm_lib/Frames and Transforms/Rigid Transform  TranslationMethod=Cartesian  TranslationLengthUnit=cm  TranslationStandardAxis=+Z  TranslationStandardOffset=0  TranslationCartesianOffset=[-0.1 -0.41 0]  TranslationROffset=0  TranslationROffsetUnits=m  TranslationZOffset=0  TranslationZOffsetUnits=m  TranslationThetaOffset=0  TranslationThetaOffsetUnits=deg  RotationMethod=None  RotationAngleUnits=deg  RotationStandardAxis=+Z  RotationAngle=16.9  RotationArbitraryAxis=[0 0 1]  FollAlignAxisA=+X  BaseAlignAxisA=+Y  FollAlignAxisB=+Y  BaseAlignAxisB=+Z  RotationSequenceAxes=FollowerAxes  RotationSequence=XYX  RotationSequenceAngles=[0 0 0]  RotationSequenceAnglesUnits=deg  RotationMatrix=[1 0 0; 0 1 0; 0 0 1]  BlockFunction=simmechanics.library.frames_transforms.rigid_transform
  ReferenceFrame : sm_lib/Frames and Transforms/Reference Frame  BlockFunction=simmechanics.library.frames_transforms.reference_frame
  Solid : sm_lib/Body Elements/Solid  InertiaType=Custom  Mass=0.10886700000000001  MassUnits=kg  CenterOfMass=[-7.0735826771653532 -5.4207086614173221 0.43749999999999994]  CenterOfMassUnits=in  MomentsOfInertia=[0.15492559985119964 0.37627255254510494 0.51721278442556873]  MomentsOfInertiaUnits=kg*in^2  ProductsOfInertia=[0 0 0.22537510075020142]  ProductsOfInertiaUnits=kg*in^2  DensityBased=on  Density=1000  DensityUnits=kg/(m^3)  DoExposeReferenceFrame=on  SerializedFrames=<Frames/>  GraphicType=FromGeometry  MarkerShape=Sphere  MarkerSize=10  MarkerSizeUnits=m  GraphicVisPropType=SimpleVisualProperties  GraphicDiffuseColor=[0.647059 0.619608 0.588235]  GraphicSpecularColor=[0.5 0.5 0.5 1.0]  GraphicAmbientColor=[0.15 0.15 0.15 1.0]  GraphicEmissiveColor=[0.0 0.0 0.0 1.0]  GraphicShininess=75  GraphicOpacity=1  GeometryShape=FromFile  RectangleSize=[1 1]  RectangleSizeUnits=m  BrickDimensions=[1 1 1]  BrickDimensionUnits=m  CylinderRadius=1  CylinderRadiusUnits=m  CylinderLength=1  CylinderLengthUnits=m  SphereRadius=1  SphereRadiusUnits=m  EllipsoidRadii=[1 1 1]  EllipsoidRadiiUnits=m  ExtrusionCrossSection=[1 1; -1 1; -1 -1; 1 -1]  ExtrusionCrossSectionUnits=m  ExtrusionLength=1  ExtrusionLengthUnits=m  PolygonNumSides=3  PolygonOuterRadius=1  PolygonOuterRadiusUnits=m  ExtGeomFileType=STL  ExtGeomFileName=ankle_rsm_2_Default_sldprt.STL  ExtGeomFileUnits=in  RevolutionCrossSection=[1 1; 1 -1; 2 -1; 2 1]  RevolutionCrossSectionUnits=m  RevolutionExtent=Full  RevolutionAngle=180  RevolutionAngleUnits=deg  BlockFunction=simmechanics.library.body_elements.solid
  Shin conn : PMIOPort  Port=1  Side=Left
  Spring conn : PMIOPort  Port=2  Side=Right
  connections:
  ReferenceFrame/RConn1 -- Ref-2-Spring/LConn1 -- Ref-2-Shin/RConn1 -- Solid/RConn1
  Ref-2-Shin/LConn1 -- Shin conn/RConn1
  Ref-2-Spring2/RConn1 -- Spring conn/RConn1
  Ref-2-Spring2/LConn1 -- Ref-2-Spring/RConn1

== system robot_leg_opt/Robotic Leg Simulator/Left Leg/Ankle pin1 ==
  Ref-2-Center : sm_lib/Frames and Transforms/Rigid Transform  TranslationMethod=Cartesian  TranslationLengthUnit=cm  TranslationStandardAxis=+Z  TranslationStandardOffset=0  TranslationCartesianOffset=[1.8 0 0]  TranslationROffset=0  TranslationROffsetUnits=m  TranslationZOffset=0  TranslationZOffsetUnits=m  TranslationThetaOffset=0  TranslationThetaOffsetUnits=deg  RotationMethod=StandardAxis  RotationAngleUnits=deg  RotationStandardAxis=+Y  RotationAngle=90  RotationArbitraryAxis=[0.57735026918962584 0.57735026918962573 0.57735026918962573]  FollAlignAxisA=+X  BaseAlignAxisA=+Y  FollAlignAxisB=+Y  BaseAlignAxisB=+Z  RotationSequenceAxes=FollowerAxes  RotationSequence=XYX  RotationSequenceAngles=[0 0 0]  RotationSequenceAnglesUnits=deg  RotationMatrix=[1 0 0; 0 1 0; 0 0 1]  BlockFunction=simmechanics.library.frames_transforms.rigid_transform
  ReferenceFrame : sm_lib/Frames and Transforms/Reference Frame  BlockFunction=simmechanics.library.frames_transforms.reference_frame
  Solid : sm_lib/Body Elements/Solid  InertiaType=Custom  Mass=0.038628200000000001  MassUnits=kg  CenterOfMass=[0.71555118110236215 0 0]  CenterOfMassUnits=in  MomentsOfInertia=[0.0013360050220100437 0.0082046624093248168 0.0082046624093248168]  MomentsOfInertiaUnits=kg*in^2  ProductsOfInertia=[0 0 0]  ProductsOfInertiaUnits=kg*in^2  DensityBased=on  Density=1000  DensityUnits=kg/(m^3)  DoExposeReferenceFrame=on  SerializedFrames=<Frames/>  GraphicType=FromGeometry  MarkerShape=Sphere  MarkerSize=10  MarkerSizeUnits=m  GraphicVisPropType=SimpleVisualProperties  GraphicDiffuseColor=[0.647059 0.619608 0.588235]  GraphicSpecularColor=[0.5 0.5 0.5 1.0]  GraphicAmbientColor=[0.15 0.15 0.15 1.0]  GraphicEmissiveColor=[0.0 0.0 0.0 1.0]  GraphicShininess=75  GraphicOpacity=1  GeometryShape=FromFile  RectangleSize=[1 1]  RectangleSizeUnits=m  BrickDimensions=[1 1 1]  BrickDimensionUnits=m  CylinderRadius=1  CylinderRadiusUnits=m  CylinderLength=1  CylinderLengthUnits=m  SphereRadius=1  SphereRadiusUnits=m  EllipsoidRadii=[1 1 1]  EllipsoidRadiiUnits=m  ExtrusionCrossSection=[1 1; -1 1; -1 -1; 1 -1]  ExtrusionCrossSectionUnits=m  ExtrusionLength=1  ExtrusionLengthUnits=m  PolygonNumSides=3  PolygonOuterRadius=1  PolygonOuterRadiusUnits=m  ExtGeomFileType=STL  ExtGeomFileName=damper_pin_Default_sldprt.STL  ExtGeomFileUnits=in  RevolutionCrossSection=[1 1; 1 -1; 2 -1; 2 1]  RevolutionCrossSectionUnits=m  RevolutionExtent=Full  RevolutionAngle=180  RevolutionAngleUnits=deg  BlockFunction=simmechanics.library.body_elements.solid
  Pin center : PMIOPort  Port=1  Side=Left
  Pin center2 : PMIOPort  Port=2  Side=Right
  connections:
  Ref-2-Center/LConn1 -- ReferenceFrame/RConn1 -- Solid/RConn1
  Pin center/RConn1 -- Ref-2-Center/RConn1 -- Pin center2/RConn1

== system robot_leg_opt/Robotic Leg Simulator/Left Leg/Body Mass ==
  ReferenceFrame : sm_lib/Frames and Transforms/Reference Frame  BlockFunction=simmechanics.library.frames_transforms.reference_frame
  Solid : sm_lib/Body Elements/Solid  InertiaType=CalculateFromGeometry  Mass=30  MassUnits=kg  CenterOfMass=[0 0 0]  CenterOfMassUnits=m  MomentsOfInertia=[1 1 1]  MomentsOfInertiaUnits=kg*m^2  ProductsOfInertia=[0 0 0]  ProductsOfInertiaUnits=kg*m^2  DensityBased=off  Density=1000  DensityUnits=kg/(m^3)  DoExposeReferenceFrame=on  SerializedFrames=<Frames/>  GraphicType=FromGeometry  MarkerShape=Sphere  MarkerSize=10  MarkerSizeUnits=m  GraphicVisPropType=SimpleVisualProperties  GraphicDiffuseColor=[0.5 0.5 0.5]  GraphicSpecularColor=[0.5 0.5 0.5 1.0]  GraphicAmbientColor=[0.15 0.15 0.15 1.0]  GraphicEmissiveColor=[0.0 0.0 0.0 1.0]  GraphicShininess=75  GraphicOpacity=1.0  GeometryShape=Sphere  RectangleSize=[1 1]  RectangleSizeUnits=m  BrickDimensions=[1 1 1]  BrickDimensionUnits=m  CylinderRadius=1  CylinderRadiusUnits=m  CylinderLength=1  CylinderLengthUnits=m  SphereRadius=0.1  SphereRadiusUnits=m  EllipsoidRadii=[1 1 1]  EllipsoidRadiiUnits=m  ExtrusionCrossSection=[1 1; -1 1; -1 -1; 1 -1]  ExtrusionCrossSectionUnits=m  ExtrusionLength=1  ExtrusionLengthUnits=m  PolygonNumSides=3  PolygonOuterRadius=1  PolygonOuterRadiusUnits=m  ExtGeomFileType=STL  ExtGeomFileUnits=m  RevolutionCrossSection=[1 1; 1 -1; 2 -1; 2 1]  RevolutionCrossSectionUnits=m  RevolutionExtent=Full  RevolutionAngle=180  RevolutionAngleUnits=deg  BlockFunction=simmechanics.library.body_elements.solid
  Mass conn : PMIOPort  Port=1  Side=Right
  connections:
  ReferenceFrame/RConn1 -- Mass conn/RConn1 -- Solid/RConn1

== system robot_leg_opt/Robotic Leg Simulator/Left Leg/Bottom Damper pin ==
  Ref-2-Center : sm_lib/Frames and Transforms/Rigid Transform  TranslationMethod=Cartesian  TranslationLengthUnit=cm  TranslationStandardAxis=+Z  TranslationStandardOffset=0  TranslationCartesianOffset=[1.8 0 0]  TranslationROffset=0  TranslationROffsetUnits=m  TranslationZOffset=0  TranslationZOffsetUnits=m  TranslationThetaOffset=0  TranslationThetaOffsetUnits=deg  RotationMethod=StandardAxis  RotationAngleUnits=deg  RotationStandardAxis=+Y  RotationAngle=90  RotationArbitraryAxis=[0.57735026918962584 0.57735026918962573 0.57735026918962573]  FollAlignAxisA=+X  BaseAlignAxisA=+Y  FollAlignAxisB=+Y  BaseAlignAxisB=+Z  RotationSequenceAxes=FollowerAxes  RotationSequence=XYX  RotationSequenceAngles=[0 0 0]  RotationSequenceAnglesUnits=deg  RotationMatrix=[1 0 0; 0 1 0; 0 0 1]  BlockFunction=simmechanics.library.frames_transforms.rigid_transform
  ReferenceFrame : sm_lib/Frames and Transforms/Reference Frame  BlockFunction=simmechanics.library.frames_transforms.reference_frame
  Solid : sm_lib/Body Elements/Solid  InertiaType=Custom  Mass=0.038628200000000001  MassUnits=kg  CenterOfMass=[0.71555118110236215 0 0]  CenterOfMassUnits=in  MomentsOfInertia=[0.0013360050220100437 0.0082046624093248168 0.0082046624093248168]  MomentsOfInertiaUnits=kg*in^2  ProductsOfInertia=[0 0 0]  ProductsOfInertiaUnits=kg*in^2  DensityBased=on  Density=1000  DensityUnits=kg/(m^3)  DoExposeReferenceFrame=on  SerializedFrames=<Frames/>  GraphicType=FromGeometry  MarkerShape=Sphere  MarkerSize=10  MarkerSizeUnits=m  GraphicVisPropType=SimpleVisualProperties  GraphicDiffuseColor=[0.647059 0.619608 0.588235]  GraphicSpecularColor=[0.5 0.5 0.5 1.0]  GraphicAmbientColor=[0.15 0.15 0.15 1.0]  GraphicEmissiveColor=[0.0 0.0 0.0 1.0]  GraphicShininess=75  GraphicOpacity=1  GeometryShape=FromFile  RectangleSize=[1 1]  RectangleSizeUnits=m  BrickDimensions=[1 1 1]  BrickDimensionUnits=m  CylinderRadius=1  CylinderRadiusUnits=m  CylinderLength=1  CylinderLengthUnits=m  SphereRadius=1  SphereRadiusUnits=m  EllipsoidRadii=[1 1 1]  EllipsoidRadiiUnits=m  ExtrusionCrossSection=[1 1; -1 1; -1 -1; 1 -1]  ExtrusionCrossSectionUnits=m  ExtrusionLength=1  ExtrusionLengthUnits=m  PolygonNumSides=3  PolygonOuterRadius=1  PolygonOuterRadiusUnits=m  ExtGeomFileType=STL  ExtGeomFileName=damper_pin_Default_sldprt.STL  ExtGeomFileUnits=in  RevolutionCrossSection=[1 1; 1 -1; 2 -1; 2 1]  RevolutionCrossSectionUnits=m  RevolutionExtent=Full  RevolutionAngle=180  RevolutionAngleUnits=deg  BlockFunction=simmechanics.library.body_elements.solid
  Pin center : PMIOPort  Port=1  Side=Left
  Pin center2 : PMIOPort  Port=2  Side=Right
  connections:
  Ref-2-Center/LConn1 -- ReferenceFrame/RConn1 -- Solid/RConn1
  Pin center/RConn1 -- Ref-2-Center/RConn1 -- Pin center2/RConn1
